simulink model "StateSpaceRepresentation"  (R2020b)
settings: Solver=VariableStepAuto  StartTime=0.0  StopTime=10.0  RelTol=1e-3
settings Model: Creator=sara6  LastModifiedBy=sara6

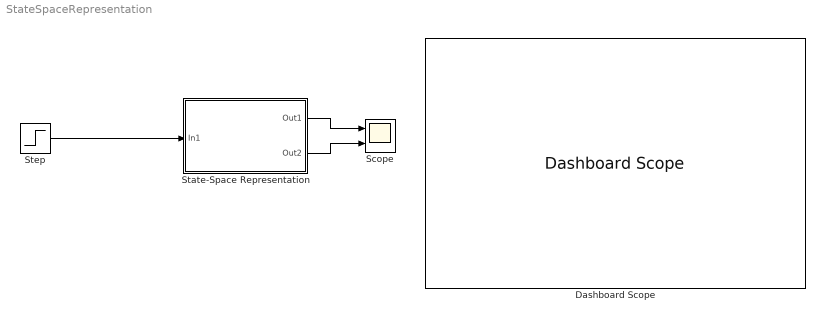
== system StateSpaceRepresentation ==
  Dashboard Scope : DashboardScope
  Scope : Scope  NumInputPorts=2
  State-Space Representation : Subsystem
  Step : Step  After=20/180*pi  SampleTime=0
  wires:
  Step/1 -> State-Space Representation/1(In1)
  State-Space Representation/1(Out1) -> Scope/1
  State-Space Representation/2(Out2) -> Scope/2

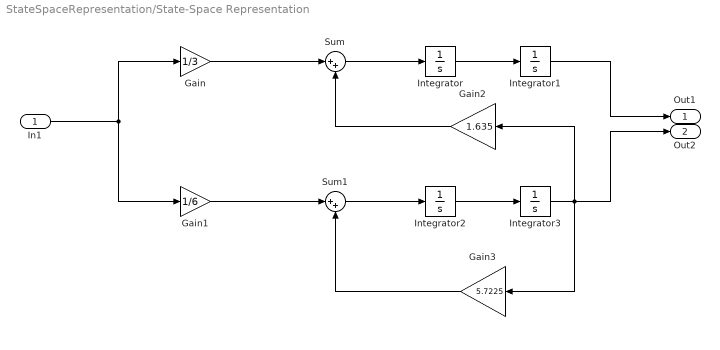
== system StateSpaceRepresentation/State-Space Representation ==
  In1 : Inport
  Gain : Gain  Gain=1/3
  Gain1 : Gain  Gain=1/6
  Gain2 : Gain  Gain=1.635
  Gain3 : Gain  Gain=5.7225
  Integrator{,1..3} (4 alike) : Integrator
  Sum : Sum  Inputs=|++
  Sum1 : Sum  Inputs=|++
  Out1 : Outport
  Out2 : Outport  Port=2
  wires:
  Integrator/1 -> Integrator1/1
  Gain3/1 -> Sum1/2
  Sum1/1 -> Integrator2/1
  Gain2/1 -> Sum/2
  Gain/1 -> Sum/1
  Gain1/1 -> Sum1/1
  Sum/1 -> Integrator/1
  Integrator3/1 -> Out2/1, Gain2/1, Gain3/1
  Integrator2/1 -> Integrator3/1
  In1/1 -> Gain/1, Gain1/1
  Integrator1/1 -> Out1/1
